simulink model "demoUDPhost"  (R2016a)
settings: Solver=FixedStepDiscrete  StartTime=0.0  StopTime=inf  FixedStep=1  RelTol=1e-3
libraries: dspnetwork x2, etargetslib x1, simulink x1
settings Model: Creator=user  LastModifiedBy=user
settings RTWCC: PackageGeneratedCodeAndArtifacts=on

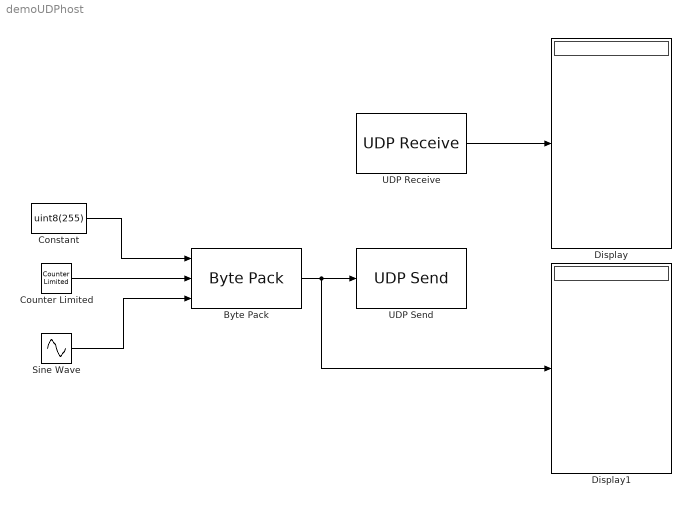
== system demoUDPhost ==
  Byte Pack : etargetslib/Byte Pack  datatypes={'uint8', 'uint8', 'double'}  byteAlign=1
  Constant : Constant  Value=uint8(255)
  Counter Limited : simulink/Sources/Counter Limited  uplimit=100  tsamp=1
  Display : Display
  Display1 : Display
  Sine Wave : Sin  SineType=Sample based  SampleTime=1
  UDP Receive : dspnetwork/UDP Receive  localURL='0.0.0.0'  localPort=25001  remoteURL='0.0.0.0'  remotePort=-1  recvBufferSize=20  dims=10  signalDatatype=uint8  isVarSize=on  showBlockingTime=on  blockingTime=1  sampletime=1  blockPlatform=HOST
  UDP Send : dspnetwork/UDP Send  remoteURL='255.255.255.255'  remotePort=25000  localURL='0.0.0.0'  localPortSource=Automatically determine  localPort=-1  sampletime=-1  blockPlatform=HOST  separateLengthPort=0
  wires:
  Byte Pack/1 -> Display1/1, UDP Send/1
  Counter Limited/1 -> Byte Pack/2
  Constant/1 -> Byte Pack/1
  Sine Wave/1 -> Byte Pack/3
  UDP Receive/1 -> Display/1
